simulink model "SimLin"  (R2016b)
settings: Solver=ode45  StartTime=0.0  StopTime=20  RelTol=1e-3  EnableMultiTasking=on
values from neighbouring files (symbols this model uses):
  IntegerTimeDelay = 2    [SetupLin.m]
  SampleTime = 0.01    [SetupHIL.m]    (also in SetupLin.m = 0.02; SetupNL.m = 0.02)
undefined symbols (not defined in the file or in its folder): linmodel, OperatingPoint, TrimCondition
undefined symbols (not defined in the file): AC
libraries: Sensors_Lib x10, simulink_extras x8, Actuator_Lib x1, simulink x1
settings Model: Creator=austinmurch  LastModifiedBy=rega0051
settings DataIOCC: LimitDataPoints=on  SaveFormat=Array  SignalLoggingSaveFormat=ModelDataLogs
settings OptimizationCC: ExpressionDepthLimit=2147483647  LifeSpan=inf  SimCompilerOptimization=on
settings DebuggingCC: UnderspecifiedInitializationDetection=Classic  MergeDetectMultiDrivingBlocksExec=none  SolverPrmCheckMsg=warning  FcnCallInpInsideContextMsg=warning  StateNameClashWarn=warning  StrictBusMsg=Warning  SFUnexpectedBacktrackingDiag=warning  SFNoUnconditionalDefaultTransitionDiag=warning  SFExecutionAtInitializationDiag=none
settings HardwareCC: ProdBitPerPointer=32  ProdBitPerSizeT=32  ProdBitPerPtrDiffT=32  ProdLargestAtomicInteger=Long  ProdLargestAtomicFloat=Double  ProdEndianess=BigEndian  ProdWordSize=32  ProdHWDeviceType=Freescale->32-bit PowerPC
settings ModelReferenceCC: PropagateSignalLabelsOutOfModel=off
settings GRTTargetCC: TargetLangStandard=C89/C90 (ANSI)  GeneratePreprocessorConditionals=Disable all  CombineOutputUpdateFcns=off  GRTInterface=on
settings ConfigComp: CovMetricSettings=dw  CovHtmlReporting=on  CovSaveCumulativeToWorkspaceVar=on  CovSaveSingleToWorkspaceVar=on  CovExternalEMLEnable=off

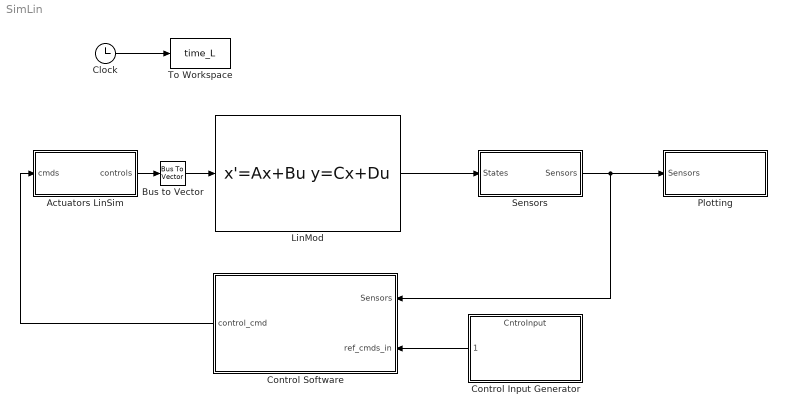
== system SimLin ==
  Actuators LinSim : Subsystem  BlockChoice=UltraStick LinSim  mask{aircraft=AC.aircraft}
      mask help: Set actuator models, either 'UltraStick120', 'UltraStick25e', or 'miniMUTT'
      mask init:
      | pathname = gcb;
      | 
      | switch lower(aircraft)
      |     case 'ultrastick120'
      |         set_param(pathname,'BlockChoice','UltraStick LinSim');
      |     case 'ultrastick25e'
      |         set_param(pathname,'BlockChoice','UltraStick LinSim');
      |     case 'minimutt'
      |         set_param(pathname,'BlockChoice','miniMUTT LinSim');
      | end
      settings: AttributesFormatString=%<BlockChoice>  TemplateBlock=Actuator_Lib/Actuators LinSim  MemberBlocks=UltraStick LinSim,miniMUTT LinSim
  Bus to Vector : BusToVector
  Clock : Clock
  Control Input Generator : ModelReference  ModelNameDialog=CntroInput  SimulationMode=Normal  ModelReferenceVersion=1.13
  Control Software : Subsystem
  LinMod : StateSpace  A=linmodel.a  B=linmodel.b  C=linmodel.c  D=linmodel.d  X0=0
  Plotting : Subsystem
  Sensors : Subsystem
  To Workspace : ToWorkspace  VariableName=time_L  SampleTime=SampleTime
  wires:
  LinMod/1 -> Sensors/1(States)
  Control Software/1(control_cmd) -> Actuators LinSim/1(cmds)
  Sensors/1(Sensors) -> Plotting/1(Sensors), Control Software/1(Sensors)
  Clock/1 -> To Workspace/1
  Control Input Generator/1 -> Control Software/2(ref_cmds_in)
  Actuators LinSim/1(controls) -> Bus to Vector/1
  Bus to Vector/1 -> LinMod/1

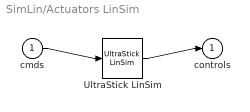
== system SimLin/Actuators LinSim ==
  cmds : Inport
  UltraStick LinSim : Actuator_Lib/UltraStick LinSim
  controls : Outport
  wires:
  cmds/1 -> UltraStick LinSim/1
  UltraStick LinSim/1 -> controls/1

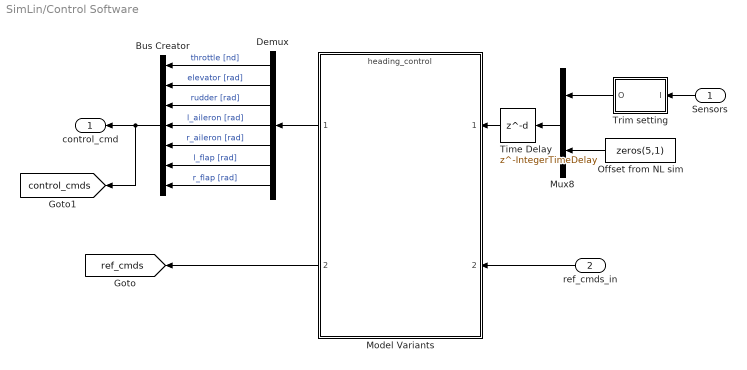
== system SimLin/Control Software ==
  Sensors : Inport
  ref_cmds_in : Inport  Port=2
  Bus Creator : BusCreator  Inputs=7
  Demux : Demux  Outputs=7
  Model Variants : ModelReference  ModelNameDialog=heading_control  SimulationMode=Normal  Variant=on  ModelReferenceVersion=1.139
      settings: AttributesFormatString=%<ActiveVariant>
  Mux8 : Mux  Inputs=2
  Offset from NL sim : Constant  Value=zeros(5,1)
  Time Delay : Delay  DelayLength=IntegerTimeDelay  InitialCondition=repmat([TrimCondition.AttitudeIni;TrimCondition.RatesIni;TrimCondition.AccelsIni;OperatingPoint.op_report.Outputs(4).y;TrimCondition.WindAxesIni;0;zeros(5,1)],[1,IntegerTimeDelay])  InputProcessing=Inherited  SampleTime=SampleTime
  "Trim setting " : Subsystem  AncestorBlock=Actuator_Lib/Trim setting
  control_cmd : Outport
  tag scope: control_cmds=global, ref_cmds=global
  wires:
  Sensors/1 -> "Trim setting "/1(I)
  ref_cmds_in/1 -> Model Variants/2
  Model Variants/2 -> [ref_cmds]
  Demux/1 -> Bus Creator/1  "throttle [nd]"
  Demux/2 -> Bus Creator/2  "elevator [rad]"
  Demux/3 -> Bus Creator/3  "rudder [rad]"
  Demux/4 -> Bus Creator/4  "l_aileron [rad]"
  Demux/5 -> Bus Creator/5  "r_aileron [rad]"
  Demux/6 -> Bus Creator/6  "l_flap [rad]"
  Demux/7 -> Bus Creator/7  "r_flap [rad]"
  Bus Creator/1 -> control_cmd/1, [control_cmds]
  "Trim setting "/1(O) -> Mux8/1
  Mux8/1 -> Time Delay/1
  Offset from NL sim/1 -> Mux8/2
  Time Delay/1 -> Model Variants/1
  Model Variants/1 -> Demux/1

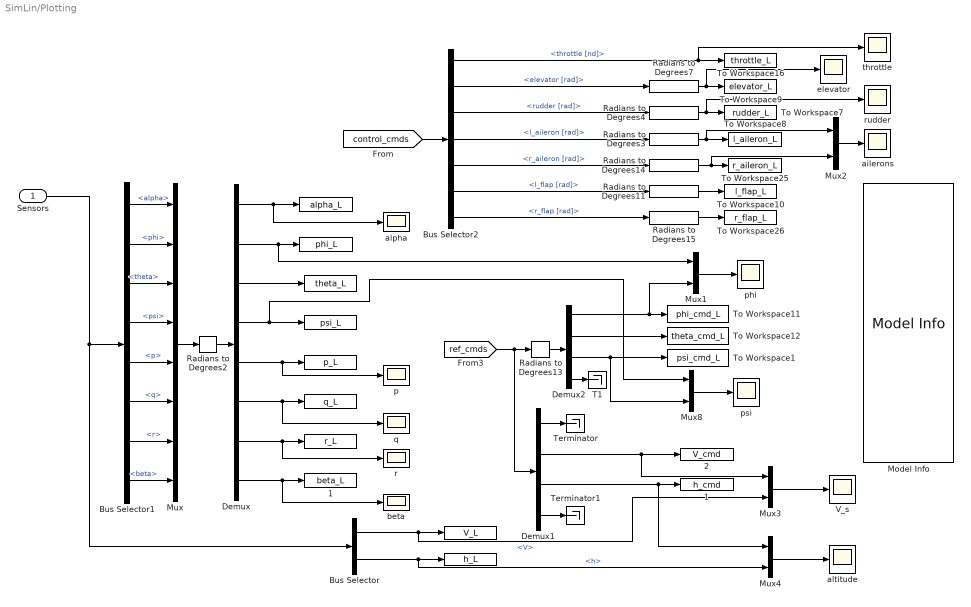
== system SimLin/Plotting ==
  Sensors : Inport
  "  " : ToWorkspace  VariableName=r_L  SampleTime=SampleTime
  "    " : ToWorkspace  VariableName=phi_L  SampleTime=SampleTime
  "      " : ToWorkspace  VariableName=theta_L  SampleTime=SampleTime
  "       " : ToWorkspace  VariableName=psi_L  SampleTime=SampleTime
  "          " : ToWorkspace  VariableName=V_L  SampleTime=SampleTime
  "           " : ToWorkspace  VariableName=p_L  SampleTime=SampleTime
  "            " : ToWorkspace  VariableName=h_L  SampleTime=SampleTime
  "                   " : ToWorkspace  VariableName=alpha_L  SampleTime=SampleTime
  "                    " : ToWorkspace  VariableName=q_L  SampleTime=SampleTime
  "                   1" : ToWorkspace  VariableName=beta_L  SampleTime=SampleTime
  "            1" : ToWorkspace  VariableName=h_cmd  SampleTime=SampleTime
  "            2" : ToWorkspace  VariableName=V_cmd  SampleTime=SampleTime
  Bus Selector : BusSelector  OutputSignals=V,h
  Bus Selector1 : BusSelector  OutputSignals=alpha,phi,theta,psi,p,q,r,beta
  Bus Selector2 : BusSelector  OutputSignals=throttle [nd],elevator [rad],rudder [rad],l_aileron [rad],r_aileron [rad],l_flap [rad],r_flap [rad]
  Demux : Demux  Outputs=8
  Demux1 : Demux  Outputs=[6 1 1 4]
  Demux2 : Demux  Outputs=[1 1 1 9]
  Model Info : simulink/Model-Wide Utilities/Model Info  BlockCM=None  Frame=on  DisplayStringWithTags=|  HorizontalTextAlignment=Center  LeftAlignmentValue=0.5  SourceBlockDiagram=SimLin  TagMaxNumber=20
      | Ref Cmd Port Info
      | 
      | 1. phi_cmd
      | 2. theta_cmd
      | 3. psi_cmd
      | 4. p_cmd
      | 5. q_cmd
      | 6. r_cmd
      | 7. V_s_cmd
      | 8. h_cmd
      | 9. gndtrk_cmd
      | 10. aoa_cmd
      | 11. aos_cmd
      | 12. gamma_cmd
      | 13. signal_0
      | 14. signal_1
      | 15. signal_2
      | 16. signal_3
      | 17. signal_4
      | 18. signal_5
      | 19. signal_6
      | 20. signal_7
      | 21. signal_8
      | 22. signal_9
  Mux : Mux  Inputs=8
  Mux{1..4,8} (5 alike) : Mux  Inputs=2
  Radians to Degrees{2..4,7,11,13..15} (8 alike) : simulink_extras/Transformations/Radians to Degrees
  T1 : Terminator
  Terminator : Terminator
  Terminator1 : Terminator
  To Workspace1 : ToWorkspace  VariableName=psi_cmd_L  SampleTime=SampleTime
  To Workspace10 : ToWorkspace  VariableName=l_flap_L  SampleTime=SampleTime
  To Workspace11 : ToWorkspace  VariableName=phi_cmd_L  SampleTime=SampleTime
  To Workspace12 : ToWorkspace  VariableName=theta_cmd_L  SampleTime=SampleTime
  To Workspace16 : ToWorkspace  VariableName=throttle_L  SampleTime=SampleTime
  To Workspace25 : ToWorkspace  VariableName=r_aileron_L  SampleTime=SampleTime
  To Workspace26 : ToWorkspace  VariableName=r_flap_L  SampleTime=SampleTime
  To Workspace7 : ToWorkspace  VariableName=rudder_L  SampleTime=SampleTime
  To Workspace8 : ToWorkspace  VariableName=l_aileron_L  SampleTime=SampleTime
  To Workspace9 : ToWorkspace  VariableName=elevator_L  SampleTime=SampleTime
  V_s : Scope
  ailerons : Scope
  alpha : Scope
  altitude : Scope
  beta : Scope
  elevator : Scope
  p : Scope
  phi : Scope
  psi : Scope
  q : Scope
  r : Scope
  rudder : Scope
  throttle : Scope
  wires:
  Sensors/1 -> Bus Selector1/1, Bus Selector/1
  Mux/1 -> Radians to Degrees2/1
  Radians to Degrees2/1 -> Demux/1
  Bus Selector1/1 -> Mux/1  "<alpha>"
  Bus Selector1/2 -> Mux/2  "<phi>"
  Bus Selector1/3 -> Mux/3  "<theta>"
  Bus Selector1/4 -> Mux/4  "<psi>"
  Bus Selector1/5 -> Mux/5  "<p>"
  Bus Selector1/6 -> Mux/6  "<q>"
  Bus Selector1/7 -> Mux/7  "<r>"
  Demux/2 -> "    "/1, Mux1/1
  Demux/3 -> "      "/1
  Demux/4 -> Mux8/1, "       "/1
  Demux/5 -> "           "/1, p/1
  Demux/6 -> "                    "/1, q/1
  Demux/7 -> "  "/1, r/1
  Radians to Degrees3/1 -> To Workspace8/1, Mux2/1
  Radians to Degrees7/1 -> To Workspace9/1, elevator/1
  Radians to Degrees4/1 -> To Workspace7/1, rudder/1
  Radians to Degrees11/1 -> To Workspace10/1
  Bus Selector2/3 -> Radians to Degrees4/1  "<rudder [rad]>"
  Bus Selector2/4 -> Radians to Degrees3/1  "<l_aileron [rad]>"
  Radians to Degrees14/1 -> To Workspace25/1, Mux2/2
  Bus Selector2/6 -> Radians to Degrees11/1  "<l_flap [rad]>"
  Mux2/1 -> ailerons/1
  Bus Selector2/7 -> Radians to Degrees15/1  "<r_flap [rad]>"
  Radians to Degrees15/1 -> To Workspace26/1
  Bus Selector2/5 -> Radians to Degrees14/1  "<r_aileron [rad]>"
  [ref_cmds] -> Radians to Degrees13/1, Demux1/1
  Radians to Degrees13/1 -> Demux2/1
  Mux1/1 -> phi/1
  Demux2/1 -> To Workspace11/1, Mux1/2
  Mux8/1 -> psi/1
  [control_cmds] -> Bus Selector2/1
  Bus Selector2/1 -> To Workspace16/1, throttle/1  "<throttle [nd]>"
  Bus Selector2/2 -> Radians to Degrees7/1  "<elevator [rad]>"
  Demux/1 -> "                   "/1, alpha/1
  Demux1/4 -> Terminator1/1
  Demux1/1 -> Terminator/1
  Demux1/3 -> "            1"/1, Mux4/1
  Demux1/2 -> "            2"/1, Mux3/1
  Bus Selector/2 -> "            "/1, Mux4/2  "<h>"
  Bus Selector/1 -> "          "/1, Mux3/2  "<V>"
  Mux3/1 -> V_s/1
  Mux4/1 -> altitude/1
  Demux2/4 -> T1/1
  Demux2/2 -> To Workspace12/1
  Demux2/3 -> To Workspace1/1, Mux8/2
  Bus Selector1/8 -> Mux/8  "<beta>"
  Demux/8 -> "                   1"/1, beta/1

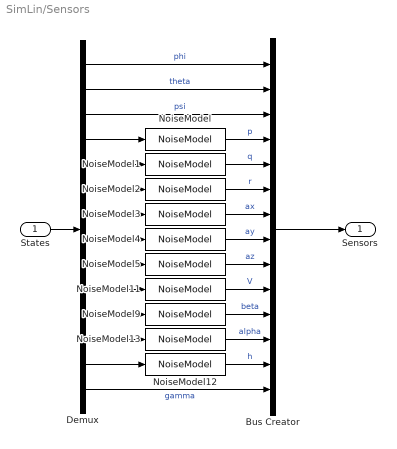
== system SimLin/Sensors ==
  States : Inport
  Bus Creator : BusCreator  Inputs=14
  Demux : Demux  Outputs=14
  NoiseModel : Sensors_Lib/NoiseModel  noise_on=AC.Sensors.NoiseOn  sigma=AC.Sensors.IMU.p_noise  seed=878230  bias=AC.Sensors.IMU.p_bias  scf=AC.Sensors.IMU.p_scf  timestep=SampleTime
  NoiseModel1 : Sensors_Lib/NoiseModel  noise_on=AC.Sensors.NoiseOn  sigma=AC.Sensors.IMU.q_noise  seed=878231  bias=AC.Sensors.IMU.q_bias  scf=AC.Sensors.IMU.q_scf  timestep=SampleTime
  NoiseModel11 : Sensors_Lib/NoiseModel  noise_on=AC.Sensors.NoiseOn  sigma=AC.Sensors.AirData.ias_noise  seed=878236  bias=AC.Sensors.AirData.ias_bias  scf=AC.Sensors.AirData.ias_scf  timestep=SampleTime
  NoiseModel12 : Sensors_Lib/NoiseModel  noise_on=AC.Sensors.NoiseOn  sigma=AC.Sensors.AirData.h_noise  seed=87828  bias=AC.Sensors.AirData.h_bias  scf=AC.Sensors.AirData.h_scf  timestep=SampleTime
  NoiseModel13 : Sensors_Lib/NoiseModel  noise_on=AC.Sensors.NoiseOn  sigma=AC.Sensors.AirData.alpha_noise  seed=87828  bias=AC.Sensors.AirData.alpha_bias  scf=AC.Sensors.AirData.alpha_scf  timestep=SampleTime
  NoiseModel2 : Sensors_Lib/NoiseModel  noise_on=AC.Sensors.NoiseOn  sigma=AC.Sensors.IMU.r_noise  seed=878232  bias=AC.Sensors.IMU.r_bias  scf=AC.Sensors.IMU.r_scf  timestep=SampleTime
  NoiseModel3 : Sensors_Lib/NoiseModel  noise_on=AC.Sensors.NoiseOn  sigma=AC.Sensors.IMU.ax_noise  seed=878233  bias=AC.Sensors.IMU.ax_bias  scf=AC.Sensors.IMU.ax_scf  timestep=SampleTime
  NoiseModel4 : Sensors_Lib/NoiseModel  noise_on=AC.Sensors.NoiseOn  sigma=AC.Sensors.IMU.ay_noise  seed=878234  bias=AC.Sensors.IMU.ay_bias  scf=AC.Sensors.IMU.ay_scf  timestep=SampleTime
  NoiseModel5 : Sensors_Lib/NoiseModel  noise_on=AC.Sensors.NoiseOn  sigma=AC.Sensors.IMU.az_noise  seed=878235  bias=AC.Sensors.IMU.az_bias  scf=AC.Sensors.IMU.az_scf  timestep=SampleTime
  NoiseModel9 : Sensors_Lib/NoiseModel  noise_on=AC.Sensors.NoiseOn  sigma=AC.Sensors.AirData.beta_noise  seed=87828  bias=AC.Sensors.AirData.beta_bias  scf=AC.Sensors.AirData.beta_scf  timestep=SampleTime
  Sensors : Outport
  wires:
  Demux/1 -> Bus Creator/1  "phi"
  Demux/2 -> Bus Creator/2  "theta"
  Demux/3 -> Bus Creator/3  "psi"
  Demux/4 -> NoiseModel/1
  Demux/5 -> NoiseModel1/1
  Demux/6 -> NoiseModel2/1
  Demux/7 -> NoiseModel3/1
  Demux/8 -> NoiseModel4/1
  Demux/9 -> NoiseModel5/1
  States/1 -> Demux/1
  Bus Creator/1 -> Sensors/1
  NoiseModel/1 -> Bus Creator/4  "p"
  NoiseModel1/1 -> Bus Creator/5  "q"
  NoiseModel2/1 -> Bus Creator/6  "r"
  NoiseModel3/1 -> Bus Creator/7  "ax"
  NoiseModel4/1 -> Bus Creator/8  "ay"
  NoiseModel5/1 -> Bus Creator/9  "az"
  Demux/10 -> NoiseModel11/1
  Demux/11 -> NoiseModel9/1
  Demux/12 -> NoiseModel13/1
  Demux/13 -> NoiseModel12/1
  NoiseModel11/1 -> Bus Creator/10  "V"
  NoiseModel13/1 -> Bus Creator/12  "alpha"
  NoiseModel9/1 -> Bus Creator/11  "beta"
  NoiseModel12/1 -> Bus Creator/13  "h"
  Demux/14 -> Bus Creator/14  "gamma"

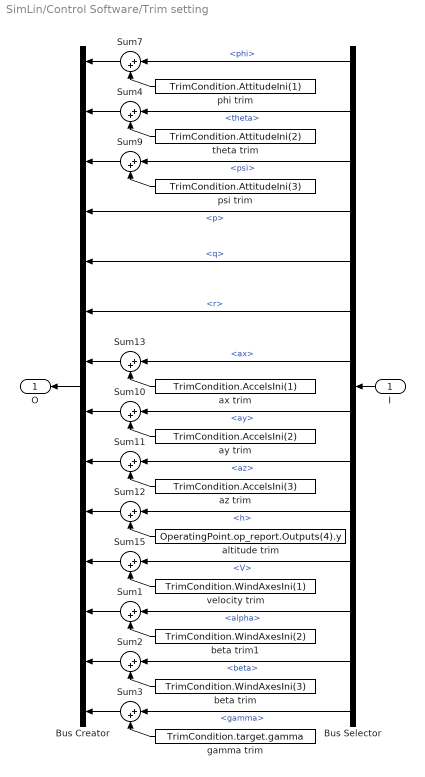
== system SimLin/Control Software/Trim setting  ==
  I : Inport
  Bus Creator : BusCreator  Inputs=14
  Bus Selector : BusSelector  OutputSignals=phi,theta,psi,p,q,r,ax,ay,az,h,V,alpha,beta,gamma
  Sum{1..4,7,9..13,15} (11 alike) : Sum  Inputs=|++
  altitude trim : Constant  Value=OperatingPoint.op_report.Outputs(4).y
  ax trim : Constant  Value=TrimCondition.AccelsIni(1)
  ay trim : Constant  Value=TrimCondition.AccelsIni(2)
  az trim : Constant  Value=TrimCondition.AccelsIni(3)
  beta trim : Constant  Value=TrimCondition.WindAxesIni(3)
  beta trim1 : Constant  Value=TrimCondition.WindAxesIni(2)
  gamma trim : Constant  Value=TrimCondition.target.gamma
  phi trim : Constant  Value=TrimCondition.AttitudeIni(1)
  psi trim : Constant  Value=TrimCondition.AttitudeIni(3)
  theta trim : Constant  Value=TrimCondition.AttitudeIni(2)
  velocity trim : Constant  Value=TrimCondition.WindAxesIni(1)
  O : Outport
  wires:
  I/1 -> Bus Selector/1
  Bus Creator/1 -> O/1
  Sum7/1 -> Bus Creator/1
  Sum9/1 -> Bus Creator/3
  Sum13/1 -> Bus Creator/7
  Sum15/1 -> Bus Creator/11
  Sum2/1 -> Bus Creator/13
  Sum1/1 -> Bus Creator/12
  Sum4/1 -> Bus Creator/2
  Bus Selector/7 -> Sum13/1  "<ax>"
  Bus Selector/1 -> Sum7/1  "<phi>"
  Bus Selector/2 -> Sum4/1  "<theta>"
  Bus Selector/3 -> Sum9/1  "<psi>"
  Bus Selector/4 -> Bus Creator/4  "<p>"
  Bus Selector/5 -> Bus Creator/5  "<q>"
  Bus Selector/6 -> Bus Creator/6  "<r>"
  Bus Selector/8 -> Sum10/1  "<ay>"
  Bus Selector/9 -> Sum11/1  "<az>"
  Bus Selector/10 -> Sum12/1  "<h>"
  Bus Selector/12 -> Sum1/1  "<alpha>"
  Bus Selector/11 -> Sum15/1  "<V>"
  Bus Selector/14 -> Sum3/1  "<gamma>"
  Bus Selector/13 -> Sum2/1  "<beta>"
  phi trim/1 -> Sum7/2
  theta trim/1 -> Sum4/2
  psi trim/1 -> Sum9/2
  Sum12/1 -> Bus Creator/10
  Sum11/1 -> Bus Creator/9
  Sum10/1 -> Bus Creator/8
  velocity trim/1 -> Sum15/2
  ax trim/1 -> Sum13/2
  ay trim/1 -> Sum10/2
  az trim/1 -> Sum11/2
  beta trim1/1 -> Sum1/2
  beta trim/1 -> Sum2/2
  altitude trim/1 -> Sum12/2
  Sum3/1 -> Bus Creator/14
  gamma trim/1 -> Sum3/2
